simulink subsystem "PowerSplitGeartrainBasic_refsub"  (R2021a)
settings: Solver=VariableStepAuto  StartTime=0.0  StopTime=10.0  RelTol=1e-3
libraries: sdl_lib x4
settings Model: Creator=isaacito  LastModifiedBy=isaacito
settings SolverCC: AlgebraicLoopSolver=TrustRegion
settings DebuggingCC: SFMachineParentedDataDiag=warning

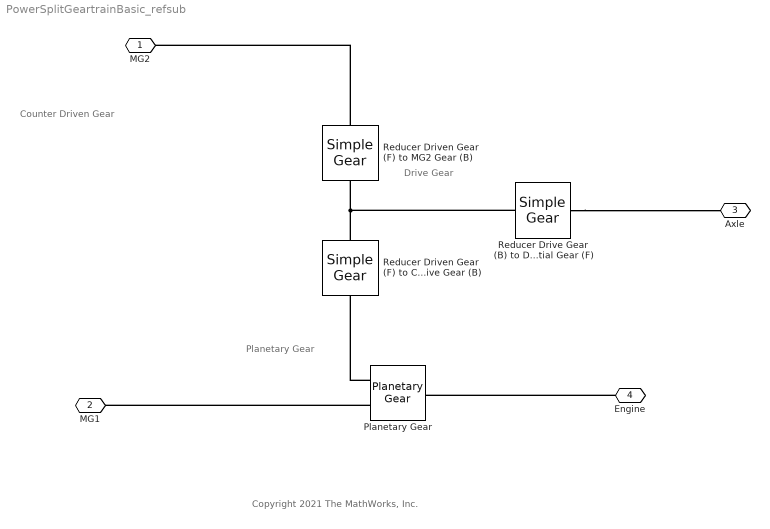
== system PowerSplitGeartrainBasic_refsub ==
  note: Copyright 2021 The MathWorks, Inc.
  note: Counter Driven Gear
  note: Drive Gear
  note: Planetary Gear
  Planetary Gear : sdl_lib/Gears/Planetary Gear  rs_ratio=powerSplit.planetary_ringToSunGearRatio  friction_model=sdl.enum.gear_friction.constant  mu_visc=powerSplit.planetary_frictions_Nm_per_rpm m*N/rpm  efficiency=powerSplit.planetary_efficiencies  temperature_TLU=[280, 300, 320] K  efficiency_sp_TLU=[.95, .9, .85]  efficiency_rp_TLU=[.95, .9, .85]  pwr_thr=smoothing.planetary_meshing_loss_thresholds_W W  thermal_mass=50 J/K  T_init=300 K  model_inertia=simscape.enum.onoff.on  planet_inertia=powerSplit.planetary_planetGearInertia_kg_m2 kg*m^2
      settings: SourceProductBaseCode=LD
  Reducer Drive Gear (B) to Differential Gear (F) : sdl_lib/Gears/Simple Gear  ratio=powerSplit.reducer_differentialGearRatio  rotation_direction=sdl.enum.shaftOutputDirection.opposite  friction_model=sdl.enum.gear_efficiencies_load.constant  mu_visc=powerSplit.reducer_friction_Nm_per_rpm N*m/(rad/s)  T_noload=0.1 N*m  T_nom=5 N*m  efficiency_nom=0.8  efficiency=powerSplit.reducer_efficiency  temperature_TLU=[280, 300, 320] K  load_TLU=[1, 5, 10] N*m  efficiency_TLU=[.95, .9, .85]  efficiency_TLU2=[.85, .8, .75; .95, .9, .85; .85, .8, .7]  w_thr=0.01 rad/s  pwr_thr=smoothing.gear_meshing_loss_threshold_W W  thermal_mass=50 J/K  enable_faults=simscape.enum.onoff.off  efficiency_fault=0.05  external_fault=simscape.enum.onoff.off  temporal_fault=simscape.enum.onoff.off  fault_time=5 s  fault_angles=pi / 12 rad  report_fault=simscape.enum.assert.action.none  temperature_specify=off  temperature_priority=High  temperature=300 K  temperature_nominal_specify=off  temperature_nominal_unit=K  temperature_nominal_value=1
  Reducer Driven Gear (F) to Counter Drive Gear (B) : sdl_lib/Gears/Simple Gear  ratio=powerSplit.reducer_counterDriveGearRatio  rotation_direction=sdl.enum.shaftOutputDirection.opposite  friction_model=sdl.enum.gear_efficiencies_load.constant  mu_visc=powerSplit.reducer_friction_Nm_per_rpm N*m/(rad/s)  T_noload=0.1 N*m  T_nom=5 N*m  efficiency_nom=0.8  efficiency=powerSplit.reducer_efficiency  temperature_TLU=[280, 300, 320] K  load_TLU=[1, 5, 10] N*m  efficiency_TLU=[.95, .9, .85]  efficiency_TLU2=[.85, .8, .75; .95, .9, .85; .85, .8, .7]  w_thr=0.01 rad/s  pwr_thr=smoothing.gear_meshing_loss_threshold_W W  thermal_mass=50 J/K  enable_faults=simscape.enum.onoff.off  efficiency_fault=0.05  external_fault=simscape.enum.onoff.off  temporal_fault=simscape.enum.onoff.off  fault_time=5 s  fault_angles=pi / 12 rad  report_fault=simscape.enum.assert.action.none  temperature_specify=off  temperature_priority=High  temperature=300 K  temperature_nominal_specify=off  temperature_nominal_unit=K  temperature_nominal_value=1
  Reducer Driven Gear (F) to MG2 Gear (B) : sdl_lib/Gears/Simple Gear  ratio=powerSplit.reducer_MG2GearRatio  rotation_direction=sdl.enum.shaftOutputDirection.opposite  friction_model=sdl.enum.gear_efficiencies_load.constant  mu_visc=powerSplit.reducer_friction_Nm_per_rpm m*N/rpm  T_noload=0.1 N*m  T_nom=5 N*m  efficiency_nom=0.8  efficiency=powerSplit.reducer_efficiency  temperature_TLU=[280, 300, 320] K  load_TLU=[1, 5, 10] N*m  efficiency_TLU=[.95, .9, .85]  efficiency_TLU2=[.85, .8, .75; .95, .9, .85; .85, .8, .7]  w_thr=0.01 rad/s  pwr_thr=smoothing.gear_meshing_loss_threshold_W W  thermal_mass=50 J/K  enable_faults=simscape.enum.onoff.off  efficiency_fault=0.05  external_fault=simscape.enum.onoff.off  temporal_fault=simscape.enum.onoff.off  fault_time=5 s  fault_angles=pi / 12 rad  report_fault=simscape.enum.assert.action.none  temperature_specify=off  temperature_priority=High  temperature=300 K  temperature_nominal_specify=off  temperature_nominal_unit=K  temperature_nominal_value=1
  MG2 : PMIOPort  Side=Left
  MG1 : PMIOPort  Port=2  Side=Left
  Axle : PMIOPort  Port=3  Side=Right
  Engine : PMIOPort  Port=4  Side=Right
  connections:
  Reducer Drive Gear (B) to Differential Gear (F)/RConn1 -- Reducer Driven Gear (F) to Counter Drive Gear (B)/RConn1 -- Reducer Driven Gear (F) to MG2 Gear (B)/RConn1
  Reducer Drive Gear (B) to Differential Gear (F)/LConn1 -- Axle/RConn1
  Planetary Gear/RConn1 -- Reducer Driven Gear (F) to Counter Drive Gear (B)/LConn1
  Engine/RConn1 -- Planetary Gear/LConn1
  Reducer Driven Gear (F) to MG2 Gear (B)/LConn1 -- MG2/RConn1
  Planetary Gear/RConn2 -- MG1/RConn1
